simulink model "proyecto_c_fc1"  (R2023b)
settings: Solver=VariableStepAuto  StartTime=0.0  StopTime=0.1  RelTol=1e-3
values from neighbouring files (symbols this model uses):
  test_fs = 10*test_FI    (= 1100000)    [simulink_parametros.m]
  test_ts = 1/test_fs    (= 9.09090909091e-07)    [simulink_parametros.m]
undefined symbols (not defined in the file or in its folder): fdesignblkfcn, gcbh, salida_sintonizador_fc1
(part 3 of 3)

== matlab function proyecto_c_fc1/MATLAB Function ==
  data: signal input; demod_am output; fs input
function demod_am = am_demodulacion(signal, fs)
    demod_am = signal .* cos(2*pi*148e3);
    % demod_am = demod(signal, 148e3, fs, 'am');
end
